simulink model "MicrostrainIMUTest02"  (R2013a)
settings: Solver=FixedStepDiscrete  StartTime=0.0  StopTime=inf  FixedStep=0.001  RelTol=1e-3
undefined symbols (not defined in the file or in its folder): IMU_Alignment_Params, KVHOrientationCal, m_XR17D15x, MicrostrainOrientationCal, standard, XOFF, XON
libraries: speedgoatlib x26, xpcethercatlib x25, xpcseriallib x13, simulink x5, dspswit3 x1, xpclib x1
(part 2 of 2)

== matlab function MicrostrainIMUTest02/Subsystem1/SerialIMU/ComputeEulerAngles ==
  data: RkIn input; wk input; RCal input; Reset input; R0In input; ZYX output; dZYX output; Rk output; R0 output; YawRolloverIn input; YawRollover output
function [ZYX, dZYX, Rk, R0, YawRollover] = fcn(RkIn, wk, RCal, Reset, R0In, YawRolloverIn) %#codegen
    % Convert from IMU frame to robot frame and compute Euler angles. The
    % yaw angle is zeroed whenever (Reset) is true.
        
    if (Reset)
        % Compute the rotation matrix which zeroes the initial yaw
        qT0 = M_to_ZYX(RkIn*RCal);
        R0  = Rz(-qT0(1));
    else
        R0 = R0In;
    end
    
    % Transform from IMU to robot frame and zero initial yaw
    Rk = R0*RkIn*RCal;
    
    % Convert Rk to ZYX Euler angles
    ZYX = M_to_ZYX(Rk);
    
    % Unroll yaw
    YawRolloverCount = YawRolloverIn(1);
    PreviousYaw      = YawRolloverIn(2);
    CurrentYaw       = ZYX(1);
    YawRolloverCount = YawRolloverCount + getYawRollover(CurrentYaw, PreviousYaw);
    YawRollover      = [YawRolloverCount; CurrentYaw];
    ZYX(1)           = ZYX(1) + 2*pi*YawRolloverCount;
    
    % Compute Euler angle derivatives
    qzT = ZYX(1);
    qyT = ZYX(2);
    
    if cos(qyT)>1e-3
        dZYX = [0 -sin(qzT) cos(qzT)*cos(qyT); 0 cos(qzT) sin(qzT)*cos(qyT); 1 0 -sin(qyT)]\(R0*RkIn*wk);
    else
        dZYX = [0; 0; 0];
    end
end

function R = Rz(t)
    R = [cos(t) -sin(t) 0; sin(t) cos(t) 0; 0 0 1];
end

function Rollover = getYawRollover(CurrentYaw, PreviousYaw)
    % Determine if a rollover has occurred on yaw angle If a rollover is
    % detected, the output Rollover is either +1 or -1, depending on the
    % direction of the rollover.
  
    if (PreviousYaw>0 && CurrentYaw < (PreviousYaw-pi))
        Rollover = 1;
    elseif (PreviousYaw<0 && CurrentYaw > (PreviousYaw+pi))
        Rollover = -1;
    else
        Rollover = 0;
    end
end

== matlab function MicrostrainIMUTest02/Subsystem1/SerialIMU/UpdateOrientation/EstimateOrientation ==
  data: DeltaAngle input; Acceleration input; Status input; Sequence input; Reset input; Rk output; wk output; Rkm1 input; wkm1 input; Akm1 input; Ak output; Seqkm1 input; Seqk output
function [Rk, wk, Ak, Seqk] = fcn(DeltaAngle,Acceleration,Status,Sequence,Reset,Rkm1,wkm1,Akm1,Seqkm1) %#codegen
    [Rk, wk, Ak, Seqk] = estimateOrientation(DeltaAngle,Acceleration,Rkm1,wkm1,Akm1,Status,Sequence,Seqkm1,Reset);
end

== matlab function MicrostrainIMUTest02/Subsystem1/SerialIMU/UpdateOrientation/MATLAB Function ==
  data: P input; Rotation output; Acceleration output; Status output; Sequence output; Temperature output; Valid output
function [Rotation,Acceleration,Status,Sequence,Temperature,Valid] = KVHParsePacket(P)
    %#codegen
    CMD = [254; 129; 255; 85]; %hex2dec(['FE';'81';'FF';'55']);
    
    Valid = false;
    if all(P(1:4) == CMD)
        Valid = kvhCheckCRC(P(1:36));
    end
    
    Rotation = parseSingle(P(5:16,:));
    Acceleration = parseSingle(P(17:28,:));
    Status = double(P(29));
    Sequence = double(P(30));
    Temperature = parseInt16(P(31:32));
end

function S = parseSingle(D)
    Stmp1 = uint32(reshape(D,4,[]));
    Stmp2 = 16777216*Stmp1(1,:) + 65536*Stmp1(2,:) + 256*Stmp1(3,:) + Stmp1(4,:);
    Stmp3 = typecast(Stmp2,'single');
    S = double(Stmp3');
end

function S = parseInt16(D)
    Stmp1 = uint16(reshape(D,2,[]));
    Stmp2 = 256*Stmp1(1,:) + Stmp1(2,:);
    S = double(Stmp2');
end

== matlab function MicrostrainIMUTest02/Subsystem/Process Orientation Matrix and Ang Rates/Convert_unit32_to_single ==
  data: u input uint32; y output single
function y = fcn(u)
%#codegen
y = typecast(u, 'single');

== matlab function MicrostrainIMUTest02/Subsystem/Process Orientation Matrix and Ang Rates/M_WI_to_ZYX_Euler_Angles ==
  data: M_RI_Params input; AngZ output; M11 input; M12 input; M13 input; M21 input; M22 input; M23 input; M31 input; M32 input; M33 input; AngY output; AngX output
function [AngZ,AngY,AngX] = fcn(M_RI_Params,M11,M12,M13,M21,M22,M23,M31,M32,M33)
%#codegen
AngZ = 0;
AngY = 0;
AngX = 0;
%Inputs are the three Euler angles (ZYX convention) in degrees which parametrize the
%matrix M_RI, and the 9 elements of the M_WI matrix reported by the IMU
M_RI_Z_rad = M_RI_Params(1)*pi/180;
M_RI_Y_rad = M_RI_Params(2)*pi/180;
M_RI_X_rad = M_RI_Params(3)*pi/180;

%Form the M_WI matrix from the inputs
M_WI = [M11,M12,M13;M21,M22,M23;M31,M32,M33];  
M_IW = M_WI.';
%Form the M_RI matrix from the paramters
M_RI = RotZ(M_RI_Z_rad)*RotY(M_RI_Y_rad)*RotX(M_RI_X_rad);
%Create the matrix that takes us from world frame 1 (z-down) to world frame
%2 (z-up)
M_W_W2 = [0 1 0;1 0 0;0 0 -1]; 

M_RW = M_IW*M_RI; %Relationship between robot frame and world frame 1 (z-down)

M_RW2 = M_W_W2*M_RW; %Relationship between robot frame and world frame 2 (z-up)

[AngX,AngY,AngZ] = M_to_ZYX(M_RW2);

end

function [AngX_out,AngY_out,AngZ_out] = M_to_ZYX(M_RW_in)
% M_to_ZYX.m
% Author: Kevin Galloway
% Date: 29AUG12
%
% Summary: This function takes a matrix (or array of matrices) M_RW_in and
% returns the Euler angles based on the ZYX convention. AngX refers to
% rotation around the X axis, AngY refers to rotation about the Y axis, and
% AngZ refers to rotation about the Z axis. If M_RW_in is an array of
% matrices (i.e. a multidimensional array), then AngX, AngY and AngZ
% will be vectors.
M31_RW_in = M_RW_in(3,1);
M32_RW_in = M_RW_in(3,2);
M33_RW_in = M_RW_in(3,3);
M21_RW_in = M_RW_in(2,1);
M11_RW_in = M_RW_in(1,1);
AngY_out = asin(-M31_RW_in);
AngX_out = atan2(M32_RW_in,M33_RW_in);
AngZ_out = atan2(M21_RW_in,M11_RW_in);
end

function M_X = RotX(phi)
M_X = [1 0 0; 0 cos(phi) -sin(phi); 0 sin(phi) cos(phi)];
end

function M_Y = RotY(theta)
M_Y = [cos(theta) 0 sin(theta); 0 1 0; -sin(theta) 0 cos(theta)];
end

function M_Z = RotZ(psi)
M_Z = [cos(psi) -sin(psi) 0; sin(psi) cos(psi) 0; 0 0 1];
end
